simulink model "test_simmetis"  (Simulink 8.0)
settings: Solver=ode45  StartTime=10  StopTime=1000  RelTol=1e-3
undefined symbols (not defined in the file): sigbuilder_block
libraries: simulink x4
settings Model: Creator=JA132999  LastModifiedBy=JA132999  ExtModeAutoUpdateStatusClock=off
settings SolverCC: AutoInsertRateTranBlk=on
settings DataIOCC: SignalLoggingSaveFormat=ModelDataLogs
settings OptimizationCC: InitFltsAndDblsToZero=on
settings DebuggingCC: SaveWithParameterizedLinksMsg=none  SignalResolutionControl=TryResolveAllWithWarning  MultiTaskDSMMsg=warning  MultiTaskCondExecSysMsg=none  FcnCallInpInsideContextMsg=UseLocalSettings  StrictBusMsg=Warning
settings RTWCC: IncludeERTFirstTime=on
settings GRTTargetCC: TargetFcnLib=ansi_tfl_tmw.mat  CombineOutputUpdateFcns=off  GRTInterface=on

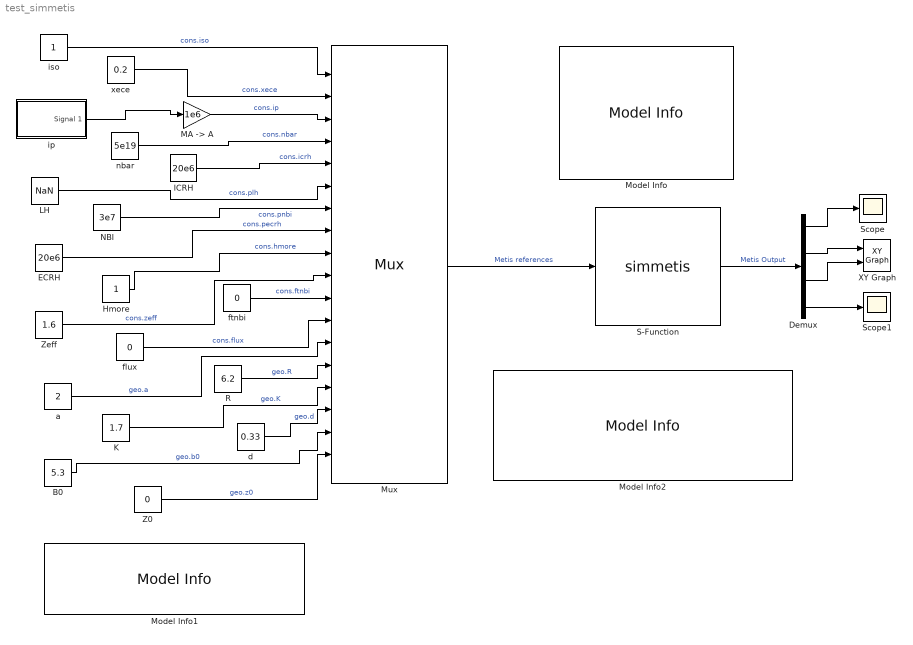
== system test_simmetis ==
  B0 : Constant  Value=5.3
  Demux : Demux
  ECRH : Constant  Value=20e6
  Hmore : Constant
  ICRH : Constant  Value=20e6
  K : Constant  Value=1.7
  LH : Constant  Value=NaN
  "MA -> A" : Gain  Gain=1e6
  Model Info : simulink/Model-Wide Utilities/Model Info  InitialBlockCM=None  BlockCM=None  Frame=on  DisplayStringWithTags=|  HorizontalTextAlignment=Center  LeftAlignmentValue=0.5  SourceBlockDiagram=test_simmetis  TagMaxNumber=20
      | SimMetis : metis sfunction interface
      | %<Created>
      | %<ModifiedBy>
      | %<ModifiedDate>
      | %<ModifiedComment>
      | %<Description>
  Model Info1 : simulink/Model-Wide Utilities/Model Info  InitialBlockCM=None  BlockCM=None  Frame=on  DisplayStringWithTags=|  HorizontalTextAlignment=Center  LeftAlignmentValue=0.5  SourceBlockDiagram=test_simmetis  TagMaxNumber=20
      | when an input is set to NaN, 
      | the correspondant reference value
      | is read from Metis file (or data) 
      | and linearely interpolate in time.
  Model Info2 : simulink/Model-Wide Utilities/Model Info  InitialBlockCM=None  BlockCM=None  Frame=on  DisplayStringWithTags=|  HorizontalTextAlignment=Left  LeftAlignmentValue=0.02  SourceBlockDiagram=test_simmetis  TagMaxNumber=20
      | Simmetis parameters :
      | * Metis_file_name : used to parametring Metis in simmetis 
      | (if empty used z0dinput in workspace,
      |  that allow to tune simulation configuration form Metis interface)
      | * list_output : cell array of output names
      | * save_file : results filename (optionnel)
      | * verbose  : if = 1 turn on information writing
  Mux : Mux  Inputs=18
      settings: DisplayOption=signals
  NBI : Constant  Value=3e7
  R : Constant  Value=6.2
  S-Function : S-Function  FunctionName=simmetis  Parameters='test_simmetis.mat',{'te0','qjli@[5,10]','pfus'},'test_save',1  EnableBusSupport=off
  Scope : Scope
      settings: YMin=25000  YMax=70000
  Scope1 : Scope
      settings: YMin=2e+07  YMax=4.75e+07
  XY Graph : simulink/Sinks/XY Graph  xmin=0.5  xmax=3  ymin=0.5  ymax=3  st=-1
  Z0 : Constant  Value=0
  Zeff : Constant  Value=1.6
  a : Constant  Value=2
  d : Constant  Value=0.33
  flux : Constant  Value=0
  ftnbi : Constant  Value=0
  ip : Subsystem  Tag=STV Subsys  LoadFcn=sigbuilder_block('load');  StartFcn=sigbuilder_block('start');  StopFcn=sigbuilder_block('stop');  ClipboardFcn=sigbuilder_block('clipboard');  mask(Sigbuilder block){}
      mask help: Sigbuilder GUI
      mask init:
      | if ~strcmp(get_param(bdroot(gcbh),'SimulationStatus'),'stopped') tuvar = sigbuilder_block('maskInit'); end
      settings: CopyFcn=sigbuilder_block('copy');  DeleteFcn=sigbuilder_block('delete');  ModelCloseFcn=sigbuilder_block('modelClose');  PreSaveFcn=sigbuilder_block('preSave');  PauseFcn=sigbuilder_block('pause')  ContinueFcn=sigbuilder_block('continue')  NameChangeFcn=sigbuilder_block('namechange');  OpenFcn=sigbuilder_block('open',[307.482 208.376 615.812 404.894 ]);  CloseFcn=sigbuilder_block('close');
      mask Display: plot(0,0,100,100,[10,10,40,40,10],[80,20,20,80,80],[40,10],[50,50], [40,27,10],[65,72,56],[40,25,25,10],[28,28,43,43]);
  iso : Constant
  nbar : Constant  Value=5e19
  xece : Constant  Value=0.2
  wires:
  Mux/1 -> S-Function/1  "Metis references"
  iso/1 -> Mux/1  "cons.iso"
  xece/1 -> Mux/2  "cons.xece"
  nbar/1 -> Mux/4  "cons.nbar"
  ip/1(Signal 1) -> "MA -> A"/1
  "MA -> A"/1 -> Mux/3  "cons.ip"
  ICRH/1 -> Mux/5  "cons.icrh"
  LH/1 -> Mux/6  "cons.plh"
  NBI/1 -> Mux/7  "cons.pnbi"
  ECRH/1 -> Mux/8  "cons.pecrh"
  Hmore/1 -> Mux/9  "cons.hmore"
  Zeff/1 -> Mux/10  "cons.zeff"
  ftnbi/1 -> Mux/11  "cons.ftnbi"
  a/1 -> Mux/13  "geo.a"
  R/1 -> Mux/14  "geo.R"
  K/1 -> Mux/15  "geo.K"
  d/1 -> Mux/16  "geo.d"
  B0/1 -> Mux/17  "geo.b0"
  Z0/1 -> Mux/18  "geo.z0"
  S-Function/1 -> Demux/1  "Metis Output"
  flux/1 -> Mux/12  "cons.flux"
  Demux/1 -> Scope/1
  Demux/4 -> Scope1/1
  Demux/2 -> XY Graph/1
  Demux/3 -> XY Graph/2

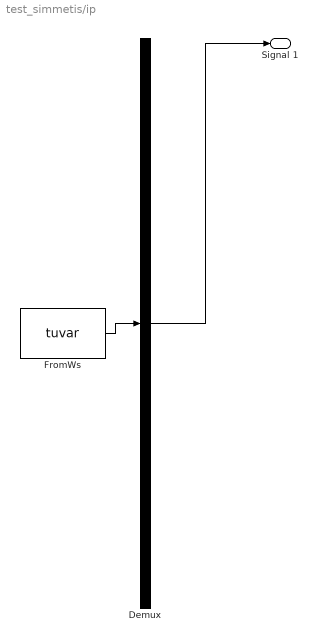
== system test_simmetis/ip ==
  Demux : Demux  Tag=STV Demux  Outputs=1
  FromWs : FromWorkspace  Tag=STV FromWs  VariableName=tuvar  SampleTime=0  SigBuilderData=DataTag0  VnvData=DataTag1
      SigBuilderData=|
      | common.afterFinalStr = 'Extrapolate'
      | common.sampleTime = 0
      | dataSet.timeRange = [0 1000]
      | dataSet.name = 'Group 1'
      | sbobj.Groups.Name = 'Group 1'
      | sbobj.Groups.Signals.Name = 'Signal 1'
      | sbobj.Groups.Signals.XData = [0 98 1000]
      | sbobj.Groups.Signals.YData = [5 15 15]
      | sbobj.Groups.TimeRange = [0 1000]
  Signal 1 : Outport  Tag=STV Outport
  wires:
  Demux/1 -> Signal 1/1
  FromWs/1 -> Demux/1
